simulink model "PraktikumSDR"  (R2023b)
settings: Solver=VariableStepAuto  StartTime=0.0  StopTime=19200*Ts  RelTol=1e-3
model workspace (MAT data in the model file):
  CodeRate = 0.75
  M = 16
  PunctureVector = [1; 1; 0; 1; 0; 1]
  TracebackDepth = 48
  Trelli.numInputSymbols = 2
  Trelli.numOutputSymbols = 4
  Trelli.numStates = 64
  Trelli.nextStates = [0  32; 0  32; 1  33; 1  33; 2  34; 2  34; 3  35; 3  35; 4  36; 4  36; 5  37; 5  37; 6  38; 6  38; 7  39; 7  39; 8  40; 8  40; 9  41; 9  41; 10  42; 10  42; 11  43; 11  43; 12  44; 12  44; 13  45; 13  45; 14  46; 14  46; 15  47; 15  47; 16  48; 16  48; 17  49; 17  49; 18  50; 18  50; 19  51; 19  51; 20  52; 20  52; 21  53; 21  53; 22  54; 22  54; 23  55; 23  55; 24  56; 24  56; 25  57; 25  57; 26  58; 26  58; 27  59; 27  59; 28  60; 28  60; 29  61; 29  61; 30  62; 30  62; 31  63; 31  63]
  Trelli.outputs = [0  3; 3  0; 1  2; 2  1; 0  3; 3  0; 1  2; 2  1; 3  0; 0  3; 2  1; 1  2; 3  0; 0  3; 2  1; 1  2; 3  0; 0  3; 2  1; 1  2; 3  0; 0  3; 2  1; 1  2; 0  3; 3  0; 1  2; 2  1; 0  3; 3  0; 1  2; 2  1; 2  1; 1  2; 3  0; 0  3; 2  1; 1  2; 3  0; 0  3; 1  2; 2  1; 0  3; 3  0; 1  2; 2  1; 0  3; 3  0; 1  2; 2  1; 0  3; 3  0; 1  2; 2  1; 0  3; 3  0; 2  1; 1  2; 3  0; 0  3; 2  1; 1  2; 3  0; 0  3]
  Ts = 5e-08
undefined symbols (not defined in the file or in its folder): doppler, get, gray, hot, j, magnitude
libraries: dspxfrm3 x12, dspobslib x11, dspstat3 x10, dspsigops x10, dspindex x7, commrflib2 x6, commcnvcod2 x6, commdigbbndam3 x6, simulink x6, commchan3 x4, dspquant2 x4, commsink2 x4
(part 1 of 3)
settings Model: Creator=suttarar@hu-berlin.de  LastModifiedBy=suttarar@hu-berlin.de

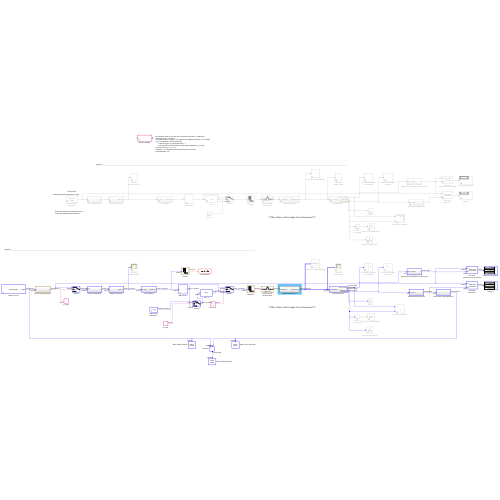
[thumbnail: Simulink's stored preview of the top-level diagram]
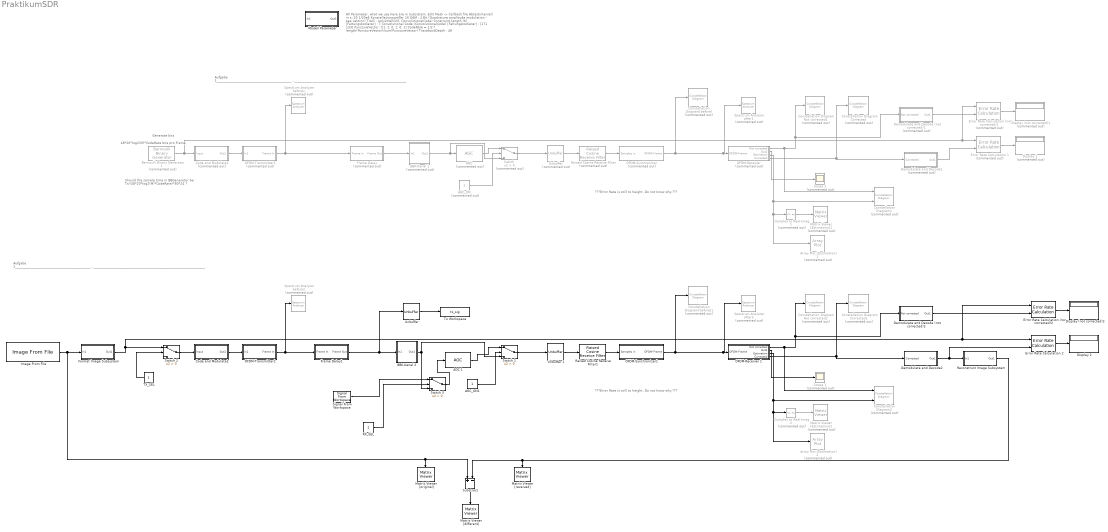
== system PraktikumSDR ==
  note: ???Error Rate is still to height. Do not know why.???
  note: Aufgabe 1______________________________________________________________________________________________________________________________________________________________________________________________________________________________________________________________________________________________________________
  note: Should the sample time in BBGenerator be:
      | Ts/(48*20*log2(M)*CodeRate)*80*24 ?
  note: All Parameter, what we use here are in Subsistem. Edit Mask -> Callback file
      | Abtastintervall in s: 20 1/20e6
      | Konstellationsgröße: 16 QAM : 4 Bit (Quadrature amplitude modulation - see Lektion)
      | Trelli : poly2trellis(K, ConvolutionalCode)
      | Constraint length (K) [Faltungskodierer] : 7
      | Convolutional Code (ConvolutionalCode) [Faltungskodierer] : [171 133]
      | PunctureVector: [[1; 1; 0; 1; 0; 1]
      | CodeRate = 1/2 * length(PunctureVector)/sum(PunctureVector)
      | TracebackDepth : 48
  note: 48*20*log2(M)*CodeRate bits pro Frame
  note: Generate bits
  note: ???Error Rate is still to height. Do not know why.???
  note: Aufgabe 2______________________________________________________________________________________________________________________________________________________________________________________________________________________________________________________________________________________________________________
  "AGC " : commrfcorlib/AGC  Commented=on  LegacyMode=off  DetectorMethod=Rectifier  LoopMethod=Linear  UpdatePeriod=100  StepSize=0.1  AdaptationStepSize=0.01  DesiredOutputPower=1  AveragingLength=16  MaximumGain=30  MaxPowerGain=10  GainOutputPort=off  InputPowerOutputPort=off  SimulateUsing=Interpreted execution
  AGC 1 : commrfcorlib/AGC  LegacyMode=off  DetectorMethod=Rectifier  LoopMethod=Linear  UpdatePeriod=100  StepSize=0.1  AdaptationStepSize=0.5  DesiredOutputPower=1  AveragingLength=16  MaximumGain=30  MaxPowerGain=10  GainOutputPort=off  InputPowerOutputPort=off  SimulateUsing=Interpreted execution
  AGC_ON : Constant  Commented=on
  AGC_ON1 : Constant
  Array Plot [Estimation]1 : ArrayPlot  Commented=on  WindowPosition=[886.000000,184.000000,800.000000,500.000000,]  ScopeFrameLocation=window  PlotAsMagnitudePhase=on  YLimits=[-0.4803 1.494]
  Array Plot [Estimation]2 : ArrayPlot  Commented=on  WindowPosition=[886.000000,184.000000,800.000000,500.000000,]  ScopeFrameLocation=window  PlotAsMagnitudePhase=on  YLimits=[-0.4803 1.494]
  BBK-Kanal 1 : Subsystem  Commented=on  mask{MaxDoppler=20, PathDelays=[0 2 5].*Ts, PathGains=[0 -16 -24], EnableMultipath=1, PathLoss=0, FrequencyOffset=50000, PhaseOffset=0, SNR=25}
      mask prompts: MaxDoppler "Dopplerverschiebung"; PathDelays "Pfadverzoergerungen"; PathGains "Pfadverstaerkungen"; EnableMultipath "SwitchBlock"; PathLoss "Pfadverlust"; FrequencyOffset "Frequenzverschiebung"; PhaseOffset "Phasenverschiebung"; SNR "AWG-Rauschen"
  BBK-Kanal 2 : Subsystem  mask{MaxDoppler=20, PathDelays=[0 2 5].*Ts, PathGains=[0 -16 -24], EnableMultipath=1, PathLoss=0, FrequencyOffset=50000, PhaseOffset=0, SNR=15}
      mask prompts: MaxDoppler "Dopplerverschiebung"; PathDelays "Pfadverzoergerungen"; PathGains "Pfadverstaerkungen"; EnableMultipath "SwitchBlock"; PathLoss "Pfadverlust"; FrequencyOffset "Frequenzverschiebung"; PhaseOffset "Phasenverschiebung"; SNR "AWG-Rauschen"
  Bernoulli Binary Generator 1 : commrandsrc3/Bernoulli Binary Generator  Commented=on  ProbabilityOfZero=0.5  SeedSource=Auto  Seed=0  SampleTime=Ts/(48*20*log2(M)*CodeRate)*80*24  SamplesPerFrame=48*20*log2(M)*CodeRate  OutputDataType=double  SimulateUsing=Interpreted execution
  Code and Modulate1 : Subsystem  Commented=on
  Code and Modulate2 : Subsystem
  Complex to Real-Imag 1 : ComplexToRealImag  Commented=on  Output=Real
  Complex to Real-Imag 2 : ComplexToRealImag  Commented=on  Output=Real
  Constellation Diagram Corrected : ConstellationDiagram  Commented=on  WindowPosition=[869.000000,188.000000,600.000000,600.000000,]  ScopeFrameLocation=window  SymbolsToDisplaySource=Property  SymbolsToDisplay=500  ReferenceConstellation="[0.70711+0.70711i        -0.70711+0.70711i        -0.70711-0.70711i         0.70711-0.70711i]"  XLimits=[-1.71,1.66]  YLimits=[-1.67,1.51]  ShowLegend=on
  Constellation Diagram Corrected1 : ConstellationDiagram  Commented=on  WindowPosition=[869.000000,188.000000,600.000000,600.000000,]  ScopeFrameLocation=window  SymbolsToDisplaySource=Property  SymbolsToDisplay=500  ReferenceConstellation="[0.70711+0.70711i        -0.70711+0.70711i        -0.70711-0.70711i         0.70711-0.70711i]"  XLimits=[-1.71,1.66]  YLimits=[-1.67,1.51]  ShowLegend=on
  Constellation Diagram Not corrected1 : ConstellationDiagram  Commented=on  WindowPosition=[922.000000,306.000000,600.000000,600.000000,]  ScopeFrameLocation=window  ReferenceConstellation="[0.70711+0.70711i        -0.70711+0.70711i        -0.70711-0.70711i         0.70711-0.70711i]"  XLimits=[-1.55,1.51]  YLimits=[-1.43,1.46]  ShowLegend=on
  Constellation Diagram Not corrected2 : ConstellationDiagram  Commented=on  WindowPosition=[922.000000,306.000000,600.000000,600.000000,]  ScopeFrameLocation=window  ReferenceConstellation="[0.70711+0.70711i        -0.70711+0.70711i        -0.70711-0.70711i         0.70711-0.70711i]"  XLimits=[-1.55,1.51]  YLimits=[-1.43,1.46]  ShowLegend=on
  Constellation Diagram1 : ConstellationDiagram  Commented=on  NumInputPorts=2  WindowPosition=[1234.000000,143.000000,600.000000,600.000000,]  ScopeFrameLocation=window  ReferenceConstellation="{[0.70711+0.70711i        -0.70711+0.70711i        -0.70711-0.70711i         0.70711-0.70711i][0.70711+0.70711i        -0.70711+0.70711i        -0.70711-0.70711i         0.70711-0.70711i]}"  XLimits=[-1.55,1.51]  YLimits=[-1.43,1.46]  ShowLegend=on
  Constellation Diagram2 : ConstellationDiagram  Commented=on  NumInputPorts=2  WindowPosition=[1234.000000,143.000000,600.000000,600.000000,]  ScopeFrameLocation=window  ReferenceConstellation="{[0.70711+0.70711i        -0.70711+0.70711i        -0.70711-0.70711i         0.70711-0.70711i][0.70711+0.70711i        -0.70711+0.70711i        -0.70711-0.70711i         0.70711-0.70711i]}"  XLimits=[-1.55,1.51]  YLimits=[-1.43,1.46]  ShowLegend=on
  Constellation Diagram[before] : ConstellationDiagram  Commented=on  WindowPosition=[219.000000,183.000000,600.000000,600.000000,]  ScopeFrameLocation=window  SymbolsToDisplaySource=Property  SymbolsToDisplay=500  ReferenceConstellation="[0.70711+0.70711i        -0.70711+0.70711i        -0.70711-0.70711i         0.70711-0.70711i]"  XLimits=[-1.71,1.66]  YLimits=[-1.67,1.51]  ShowLegend=on
  Constellation Diagram[before]1 : ConstellationDiagram  Commented=on  WindowPosition=[219.000000,183.000000,600.000000,600.000000,]  ScopeFrameLocation=window  SymbolsToDisplaySource=Property  SymbolsToDisplay=500  ReferenceConstellation="[0.70711+0.70711i        -0.70711+0.70711i        -0.70711-0.70711i         0.70711-0.70711i]"  XLimits=[-1.71,1.66]  YLimits=[-1.67,1.51]  ShowLegend=on
  Demodulate and Decode (not corrected)1 : Subsystem  Commented=on
  Demodulate and Decode (not corrected)2 : Subsystem
  Demodulate and Decode1 : Subsystem  Commented=on
  Demodulate and Decode2 : Subsystem
  Display (not corrected)1 : Display  Commented=on
  Display (not corrected)2 : Display
  Display 1 : Display  Commented=on
  Display 2 : Display
  Error Rate Calculation (not corrected)1 : commsink2/Error Rate Calculation  Commented=on  N=TracebackDepth  st_delay=48*20*log2(M)*CodeRate  cp_mode=Entire frame  subframe=[]  PMode=Port  WsName=ErrorVec  RsMode2=off  stop=off  numErr=100  maxBits=1e6
  Error Rate Calculation (not corrected)2 : commsink2/Error Rate Calculation  N=TracebackDepth  st_delay=48*20*log2(M)*CodeRate  cp_mode=Entire frame  subframe=[]  PMode=Port  WsName=ErrorVec  RsMode2=off  stop=off  numErr=100  maxBits=1e6
  Error Rate Calculation 1 : commsink2/Error Rate Calculation  Commented=on  N=TracebackDepth+2880  st_delay=0  cp_mode=Entire frame  subframe=[]  PMode=Port  WsName=ErrorVec  RsMode2=off  stop=off  numErr=100  maxBits=1e6
  Error Rate Calculation 2 : commsink2/Error Rate Calculation  N=TracebackDepth+2880  st_delay=0  cp_mode=Entire frame  subframe=[]  PMode=Port  WsName=ErrorVec  RsMode2=off  stop=off  numErr=100  maxBits=1e6
  Format Image Subsystem : Subsystem
  Frame Delay : Subsystem  Commented=on
  Frame Delay1 : Subsystem
  Image From File : visionsources/Image From File  Tag=vipblks_nd  FileName=/vol/cs-hu/suttarar/hu-home/simulink_bbk/Praktikum12/Praktikum12_Dateien (1)/grayscale.jpg  Ts=2880*10*Ts/(48*20*log2(M)*CodeRate)*80*24  imagePorts=One multidimensional signal  OutPortLabels=R|G|B  ImageDataType=Inherit from input image  sdImageDataType=uint(8)  Signed=on  WordLength=16  FractionLengthMode=User-defined  FractionLength=15
  Matrix Viewer [Estimation]1 : dspobslib/Matrix Viewer  Commented=on  ImageParams=off  CMapStr=gray(256)  AxisColorbar=on  AxisParams=off  AxisOrigin=Upper left corner  AxisTickMode=Auto  XTickRange=[0 1]  YTickRange=[0 1]  XLabel=X-axis  YLabel=Y-axis  ZLabel=Z-axis  FigPos=get(0,'defaultfigureposition')  AxisZoom=off
      settings: YMin=0.99546  YMax=1.0044
  Matrix Viewer [Estimation]2 : dspobslib/Matrix Viewer  Commented=on  ImageParams=off  CMapStr=gray(256)  AxisColorbar=on  AxisParams=off  AxisOrigin=Upper left corner  AxisTickMode=Auto  XTickRange=[0 1]  YTickRange=[0 1]  XLabel=X-axis  YLabel=Y-axis  ZLabel=Z-axis  FigPos=get(0,'defaultfigureposition')  AxisZoom=off
      settings: YMin=0.99546  YMax=1.0044
  Matrix Viewer [different] : dspobslib/Matrix Viewer  ImageParams=off  CMapStr=gray(256)  AxisColorbar=on  AxisParams=off  AxisOrigin=Upper left corner  AxisTickMode=Auto  XTickRange=[0 1]  YTickRange=[0 1]  XLabel=X-axis  YLabel=Y-axis  ZLabel=Z-axis  FigPos=get(0,'defaultfigureposition')  AxisZoom=off
      settings: YMin=0  YMax=255
  Matrix Viewer [original] : dspobslib/Matrix Viewer  ImageParams=off  CMapStr=gray(256)  AxisColorbar=on  AxisParams=off  AxisOrigin=Upper left corner  AxisTickMode=Auto  XTickRange=[0 1]  YTickRange=[0 1]  XLabel=X-axis  YLabel=Y-axis  ZLabel=Z-axis  FigPos=get(0,'defaultfigureposition')  AxisZoom=off
      settings: YMin=0  YMax=255
  Matrix Viewer [received] : dspobslib/Matrix Viewer  ImageParams=off  CMapStr=gray(256)  AxisColorbar=on  AxisParams=off  AxisOrigin=Upper left corner  AxisTickMode=Auto  XTickRange=[0 1]  YTickRange=[0 1]  XLabel=X-axis  YLabel=Y-axis  ZLabel=Z-axis  FigPos=get(0,'defaultfigureposition')  AxisZoom=off
      settings: YMin=0  YMax=255
  Modell Parameter : Subsystem  mask{Ts=1/20e6, M=16, Trelli=poly2trellis(7, [171 133]), PunctureVector=[1; 1; 0; 1; 0; 1], CodeRate=0.75, TracebackDepth=48}
      mask prompts: Ts "Abtastintervall in s"; M "Konstellationsgröße"
  "OFDM-Receiver " : Subsystem  Commented=on
  OFDM-Receiver 1 : Subsystem
  OFDM-Synchronizer : Subsystem  Commented=on
  OFDM-Synchronizer1 : Subsystem
  OFDM-Transmitter1 : Subsystem  Commented=on
  OFDM-Transmitter2 : Subsystem
  RX_SEL : Constant
  Raised Cosine Receive Filter : commfilt2/Raised Cosine Receive Filter  Commented=on  filtType=Square root  R=0.2  filtSpan=10  N=2  downFactor=2  downOffset=0  filterGain=1  RateOptions=Allow multirate processing  framing=Mute  checkCoeff=off  variableName=rcRxFilt  currentFiltSpan=10  D=5  inputOffset=0  sampMode=Mute  saveAsFlag=0  rateMode=Downsampling  checkGain=Normalized  launchFVT=on  roundingMode=Floor  overflowMode=off  coeffDataTypeStr=Inherit: Same word length as input  coeffMin=[]  coeffMax=[]  coeffLastDataTypeStr=Inherit: Same word length as input  accumDataTypeStr=Inherit: Same as product output  accumLastDataTypeStr=Inherit: Same as product output  outputDataTypeStr=Inherit: Same as accumulator  outputMin=[]  outputMax=[]  outputLastDataTypeStr=Inherit: Same as accumulator
      settings: LibrarySourceBlock=|
      | commhdlfilt/Raised Cosine
      | Receive Filter
  Raised Cosine Receive Filter1 : commfilt2/Raised Cosine Receive Filter  filtType=Square root  R=0.2  filtSpan=10  N=2  downFactor=2  downOffset=0  filterGain=1  RateOptions=Allow multirate processing  framing=Mute  checkCoeff=off  variableName=rcRxFilt1  currentFiltSpan=10  D=5  inputOffset=0  sampMode=Mute  saveAsFlag=0  rateMode=Downsampling  checkGain=Normalized  launchFVT=on  roundingMode=Floor  overflowMode=off  coeffDataTypeStr=Inherit: Same word length as input  coeffMin=[]  coeffMax=[]  coeffLastDataTypeStr=Inherit: Same word length as input  accumDataTypeStr=Inherit: Same as product output  accumLastDataTypeStr=Inherit: Same as product output  outputDataTypeStr=Inherit: Same as accumulator  outputMin=[]  outputMax=[]  outputLastDataTypeStr=Inherit: Same as accumulator
      settings: LibrarySourceBlock=|
      | commhdlfilt/Raised Cosine
      | Receive Filter
  Reconstruct Image Subsystem : Subsystem
  Scope 1 : Scope  Commented=on
  Scope 2 : Scope  Commented=on
  Signal From Workspace : dspsrcs4/Signal From Workspace  X=rx_sig  Ts=Ts/4  nsamps=7680  OutputAfterFinalValue=Setting to zero  ignoreOrWarnInputAndFrameLengths=off  OutputFrames=off
  Spectrum Analyzer after1 : SpectrumAnalyzer  Commented=on  WindowPosition=[940.000000,172.000000,800.000000,500.000000,]  ScopeFrameLocation=window  Span=20000000  StartFrequency=-10000000  StopFrequency=10000000  YLimits=[-26.81296668,18.83014348]
  Spectrum Analyzer after2 : SpectrumAnalyzer  Commented=on  WindowPosition=[940.000000,172.000000,800.000000,500.000000,]  Visible=on  ScopeFrameLocation=window  Span=20000000  StartFrequency=-10000000  StopFrequency=10000000  YLimits=[-28.40563685,17.66109951]
  Spectrum Analyzer before1 : SpectrumAnalyzer  Commented=on  WindowPosition=[6.000000,502.000000,800.000000,500.000000,]  ScopeFrameLocation=window  Span=20000000  StartFrequency=-10000000  StopFrequency=10000000  YLimits=[-24.45122434,14.99996905]
  Spectrum Analyzer before2 : SpectrumAnalyzer  Commented=on  WindowPosition=[-21.000000,360.000000,800.000000,500.000000,]  ScopeFrameLocation=window  Span=20000000  StartFrequency=-10000000  StopFrequency=10000000  YLimits=[-26.72428692,14.41237789]
  Substract : Sum  Inputs=+-
  "Switch " : Switch  Commented=on  Criteria=u2 > Threshold  SaturateOnIntegerOverflow=off  InputSameDT=off
  Switch 1 : Switch  Criteria=u2 > Threshold  SaturateOnIntegerOverflow=off  InputSameDT=off
  Switch 2 : Switch  Criteria=u2 > Threshold  SaturateOnIntegerOverflow=off  InputSameDT=off
  Switch 3 : Switch  Criteria=u2 > Threshold  SaturateOnIntegerOverflow=off  InputSameDT=off
  TX_SEL : Constant
  To Workspace : ToWorkspace  VariableName=tx_sig  SampleTime=-1
      settings: MaxDataPoints=76800  Save2DSignal=2-D array (concatenate along first dimension)
  Unbuffer : Unbuffer
  "Unbuffer " : Unbuffer  Commented=on
  Unbuffer 1 : Unbuffer
  wires:
  "OFDM-Receiver "/1(Not corrected) -> Constellation Diagram1/1, Demodulate and Decode (not corrected)1/1(Not corrected), Constellation Diagram Not corrected1/1
  Code and Modulate1/1(Out1) -> OFDM-Transmitter1/1(In1)
  Complex to Real-Imag 1/1 -> Matrix Viewer [Estimation]1/1
  "OFDM-Receiver "/2(Out2) -> Scope 2/1
  "OFDM-Receiver "/4(Corrected) -> Demodulate and Decode1/1(Corrected), Constellation Diagram Corrected/1
  Error Rate Calculation 1/1 -> Display 1/1
  Error Rate Calculation (not corrected)1/1 -> Display (not corrected)1/1
  Demodulate and Decode (not corrected)1/1(Out1) -> Error Rate Calculation (not corrected)1/2
  Demodulate and Decode1/1(Out1) -> Error Rate Calculation 1/2
  Bernoulli Binary Generator 1/1 -> Error Rate Calculation (not corrected)1/1, Error Rate Calculation 1/1, Code and Modulate1/1(Input)
  "OFDM-Receiver "/3(Estimation) -> Constellation Diagram1/2, Array Plot [Estimation]1/1, Complex to Real-Imag 1/1
  BBK-Kanal 1/1(Out1) -> "Switch "/3, "AGC "/1
  "Switch "/1 -> "Unbuffer "/1
  "AGC "/1 -> "Switch "/1
  AGC_ON/1 -> "Switch "/2
  OFDM-Synchronizer/1(OFDM-Frame) -> Spectrum Analyzer after1/1, "OFDM-Receiver "/1(OFDM-Frame), Constellation Diagram[before]/1
  "Unbuffer "/1 -> Raised Cosine Receive Filter/1
  Frame Delay/1(Frame Out) -> BBK-Kanal 1/1(In1)
  Raised Cosine Receive Filter/1 -> OFDM-Synchronizer/1(Samples in)
  OFDM-Transmitter1/1(Frame In) -> Frame Delay/1(Frame In), Spectrum Analyzer before1/1
  AGC 1/1 -> Switch 1/1
  Error Rate Calculation 2/1 -> Display 2/1
  Frame Delay1/1(Frame Out) -> Unbuffer/1, BBK-Kanal 2/1(In1)
  OFDM-Receiver 1/2(Out2) -> Scope 1/1
  Raised Cosine Receive Filter1/1 -> OFDM-Synchronizer1/1(Samples in)
  OFDM-Receiver 1/1(Not corrected) -> Constellation Diagram2/1, Demodulate and Decode (not corrected)2/1(Not corrected), Constellation Diagram Not corrected2/1
  OFDM-Receiver 1/4(Corrected) -> Demodulate and Decode2/1(Corrected), Constellation Diagram Corrected1/1
  Code and Modulate2/1(Out1) -> OFDM-Transmitter2/1(In1)
  OFDM-Receiver 1/3(Estimation) -> Constellation Diagram2/2, Array Plot [Estimation]2/1, Complex to Real-Imag 2/1
  Demodulate and Decode (not corrected)2/1(Out1) -> Error Rate Calculation (not corrected)2/2
  Error Rate Calculation (not corrected)2/1 -> Display (not corrected)2/1
  OFDM-Transmitter2/1(Frame In) -> Frame Delay1/1(Frame In), Spectrum Analyzer before2/1
  BBK-Kanal 2/1(Out1) -> Switch 3/3, Switch 1/3
  Demodulate and Decode2/1(Out1) -> Reconstruct Image Subsystem/1(In1), Error Rate Calculation 2/2
  Complex to Real-Imag 2/1 -> Matrix Viewer [Estimation]2/1
  AGC_ON1/1 -> Switch 1/2
  OFDM-Synchronizer1/1(OFDM-Frame) -> Spectrum Analyzer after2/1, OFDM-Receiver 1/1(OFDM-Frame), Constellation Diagram[before]1/1
  Switch 1/1 -> Unbuffer 1/1
  Unbuffer 1/1 -> Raised Cosine Receive Filter1/1
  Substract/1 -> Matrix Viewer [different]/1
  Format Image Subsystem/1(Out1) -> Switch 2/1, Error Rate Calculation (not corrected)2/1, Error Rate Calculation 2/1
  TX_SEL/1 -> Switch 2/2
  Switch 2/1 -> Code and Modulate2/1(Input)
  Image From File/1 -> Substract/1, Matrix Viewer [original]/1, Format Image Subsystem/1(In1)
  Reconstruct Image Subsystem/1(Out1) -> Substract/2, Matrix Viewer [received]/1
  Unbuffer/1 -> To Workspace/1
  Signal From Workspace/1 -> Switch 3/1
  RX_SEL/1 -> Switch 3/2
  Switch 3/1 -> AGC 1/1

== system PraktikumSDR/BBK-Kanal 1 ==
  In1 : Inport
  AWGN Channel : commchan3/AWGN Channel  LegacyMode=off  NoiseMethod="Signal to noise ratio  (SNR)"  noiseMode="Signal to noise ratio  (SNR)"  EbNo=10  EsNo=10  SNR=SNR  BitsPerSymbol=1  SignalPower=1  SamplesPerSymbol=1  SymbolPeriod=1  VarianceSource=Parameter  Variance=1  RandomStream=Global stream  Seed=67  SimulateUsing=Code generation
  Constant : Constant  Value=EnableMultipath
  Free Space Path Loss : commrflib2/Free Space Path Loss  mode=Decibels  dB=PathLoss  d=0.100  fc=1920
  Phase/ Frequency Offset : commrflib2/Phase// Frequency Offset  phaseOffset=PhaseOffset  freqPort=off  freqOffset=FrequencyOffset
      settings: LibrarySourceBlock=|
      | commrfcorlib/Phase//
      | Frequency
      | Offset
  SISO Fading Channel : commchan3/SISO Fading Channel  InheritSampleRate=on  SampleRate=1  PathDelays=PathDelays  AveragePathGains=PathGains  NormalizePathGains=on  FadingDistribution=Rayleigh  KFactor=3  DirectPathDopplerShift=0  DirectPathInitialPhase=0  MaximumDopplerShift=MaxDoppler  DopplerSpectrum=doppler('Jakes')  RandomStream=mt19937ar with seed  Seed=73  PathGainsOutputPort=off  ChannelFilterDelayOutputPort=off  SimulateUsing=Interpreted execution  Visualization=Off  PathsForDopplerDisplay=1  SamplesToDisplay=25%
  Switch : Switch  Criteria=u2 > Threshold  SaturateOnIntegerOverflow=off  InputSameDT=off
  Out1 : Outport
  wires:
  Phase/ Frequency Offset/1 -> AWGN Channel/1
  Free Space Path Loss/1 -> Phase/ Frequency Offset/1
  AWGN Channel/1 -> Out1/1
  Switch/1 -> Free Space Path Loss/1
  SISO Fading Channel/1 -> Switch/1
  In1/1 -> Switch/3, SISO Fading Channel/1
  Constant/1 -> Switch/2

== system PraktikumSDR/BBK-Kanal 2 ==
  In1 : Inport
  AWGN Channel : commchan3/AWGN Channel  LegacyMode=off  NoiseMethod="Signal to noise ratio  (SNR)"  noiseMode="Signal to noise ratio  (SNR)"  EbNo=10  EsNo=10  SNR=SNR  BitsPerSymbol=1  SignalPower=1  SamplesPerSymbol=1  SymbolPeriod=1  VarianceSource=Parameter  Variance=1  RandomStream=Global stream  Seed=67  SimulateUsing=Code generation
  Constant : Constant  Value=EnableMultipath
  Free Space Path Loss : commrflib2/Free Space Path Loss  mode=Decibels  dB=PathLoss  d=0.100  fc=1920
  Phase/ Frequency Offset : commrflib2/Phase// Frequency Offset  phaseOffset=PhaseOffset  freqPort=off  freqOffset=FrequencyOffset
      settings: LibrarySourceBlock=|
      | commrfcorlib/Phase//
      | Frequency
      | Offset
  SISO Fading Channel : commchan3/SISO Fading Channel  InheritSampleRate=on  SampleRate=1  PathDelays=PathDelays  AveragePathGains=PathGains  NormalizePathGains=on  FadingDistribution=Rayleigh  KFactor=3  DirectPathDopplerShift=0  DirectPathInitialPhase=0  MaximumDopplerShift=MaxDoppler  DopplerSpectrum=doppler('Jakes')  RandomStream=mt19937ar with seed  Seed=73  PathGainsOutputPort=off  ChannelFilterDelayOutputPort=off  SimulateUsing=Interpreted execution  Visualization=Off  PathsForDopplerDisplay=1  SamplesToDisplay=25%
  Switch : Switch  Criteria=u2 > Threshold  SaturateOnIntegerOverflow=off  InputSameDT=off
  Out1 : Outport
  wires:
  Phase/ Frequency Offset/1 -> AWGN Channel/1
  Free Space Path Loss/1 -> Phase/ Frequency Offset/1
  AWGN Channel/1 -> Out1/1
  Switch/1 -> Free Space Path Loss/1
  SISO Fading Channel/1 -> Switch/1
  In1/1 -> Switch/3, SISO Fading Channel/1
  Constant/1 -> Switch/2

== system PraktikumSDR/Code and Modulate1 ==
  note: Modulation
  note: Faltungscodierer
  Input : Inport
  "Convolutional Encoder " : commcnvcod2/Convolutional Encoder  trellis=Trelli  opMode=Continuous  DelayedResetAction=off  hasIniStPort=off  hasFinStPort=off  usePuncVector=on  punctureVector=PunctureVector  reset=Unused parameter value
  "Rectangular QAM Modulator Baseband " : commdigbbndam3/Rectangular QAM Modulator Baseband  M=M  InType=Bit  Enc=Gray  Mapping=[0:15]  PowType=Average Power  MinDist=2  AvgPow=1  PeakPow=1  Ph=0  outDtype=double  outWordLen=16  outUDDataType=sfix(16)  outFracLenMode=Best precision  outFracLen=15  outDataTypeStr=double  outLastDataTypeStr=double
  Out1 : Outport
  wires:
  "Convolutional Encoder "/1 -> "Rectangular QAM Modulator Baseband "/1
  "Rectangular QAM Modulator Baseband "/1 -> Out1/1
  Input/1 -> "Convolutional Encoder "/1

== system PraktikumSDR/Code and Modulate2 ==
  note: Modulation
  note: Faltungscodierer
  Input : Inport
  "Convolutional Encoder " : commcnvcod2/Convolutional Encoder  trellis=Trelli  opMode=Continuous  DelayedResetAction=off  hasIniStPort=off  hasFinStPort=off  usePuncVector=on  punctureVector=PunctureVector  reset=Unused parameter value
  "Rectangular QAM Modulator Baseband " : commdigbbndam3/Rectangular QAM Modulator Baseband  M=M  InType=Bit  Enc=Gray  Mapping=[0:15]  PowType=Average Power  MinDist=2  AvgPow=1  PeakPow=1  Ph=0  outDtype=double  outWordLen=16  outUDDataType=sfix(16)  outFracLenMode=Best precision  outFracLen=15  outDataTypeStr=double  outLastDataTypeStr=double
  Out1 : Outport
  wires:
  "Convolutional Encoder "/1 -> "Rectangular QAM Modulator Baseband "/1
  "Rectangular QAM Modulator Baseband "/1 -> Out1/1
  Input/1 -> "Convolutional Encoder "/1

== system PraktikumSDR/Demodulate and Decode (not corrected)1 ==
  Not corrected : Inport
  "Data Type Conversion " : DataTypeConversion  SaturateOnIntegerOverflow=off  RndMeth=Floor
  "Gain " : Gain  Gain=-1
  "Rectangular QAM Demodulator Baseband " : commdigbbndam3/Rectangular QAM Demodulator Baseband  M=M  OutType=Bit  DecType=Approximate log-likelihood ratio  VarSource=Dialog  Variance=1  Dec=Gray  Mapping=[0:15]  PowType=Average Power  MinDist=2  AvgPow=1  PeakPow=1  Ph=0  outDtype1=Inherit via internal rule  outDtype2=Inherit via internal rule  derotateFactorWordLen=16  derotateFactorDataTypeStr=Inherit: Same word length as input  derotateFactorLastDataTypeStr=Inherit: Same word length as input  denormFactorWordLen=16  denormFactorDataTypeStr=Inherit: Same word length as input  denormFactorLastDataTypeStr=Inherit: Same word length as input  prodOutWordLen=32  prodOutOverflowMode=Wrap  prodOutRoundingMode=Floor  prodOutOvFlMode=off  prodOutOvFlModeLastStrValue=off  sumWordLen=32
  "Uniform Encoder " : dspquant2/Uniform Encoder  peak=1  bits=4  otype=Unsigned integer
  "Viterbi Decoder " : commcnvcod2/Viterbi Decoder  trellis=Trelli  isPunctured=on  punctureVector=PunctureVector  erasures=off  dectype=Soft decision  nsdecb=4  runSigValErrCheck=off  tbdepth=TracebackDepth  opmode=Continuous  reset=off  delayedResetAction=off  smWordLength=16  outDataType=double
  Out1 : Outport
  wires:
  "Uniform Encoder "/1 -> "Data Type Conversion "/1
  "Gain "/1 -> "Uniform Encoder "/1
  "Data Type Conversion "/1 -> "Viterbi Decoder "/1
  "Rectangular QAM Demodulator Baseband "/1 -> "Gain "/1
  Not corrected/1 -> "Rectangular QAM Demodulator Baseband "/1
  "Viterbi Decoder "/1 -> Out1/1

== system PraktikumSDR/Demodulate and Decode (not corrected)2 ==
  Not corrected : Inport
  "Data Type Conversion " : DataTypeConversion  SaturateOnIntegerOverflow=off  RndMeth=Floor
  "Gain " : Gain  Gain=-1
  "Rectangular QAM Demodulator Baseband " : commdigbbndam3/Rectangular QAM Demodulator Baseband  M=M  OutType=Bit  DecType=Approximate log-likelihood ratio  VarSource=Dialog  Variance=1  Dec=Gray  Mapping=[0:15]  PowType=Average Power  MinDist=2  AvgPow=1  PeakPow=1  Ph=0  outDtype1=Inherit via internal rule  outDtype2=Inherit via internal rule  derotateFactorWordLen=16  derotateFactorDataTypeStr=Inherit: Same word length as input  derotateFactorLastDataTypeStr=Inherit: Same word length as input  denormFactorWordLen=16  denormFactorDataTypeStr=Inherit: Same word length as input  denormFactorLastDataTypeStr=Inherit: Same word length as input  prodOutWordLen=32  prodOutOverflowMode=Wrap  prodOutRoundingMode=Floor  prodOutOvFlMode=off  prodOutOvFlModeLastStrValue=off  sumWordLen=32
  "Uniform Encoder " : dspquant2/Uniform Encoder  peak=1  bits=4  otype=Unsigned integer
  "Viterbi Decoder " : commcnvcod2/Viterbi Decoder  trellis=Trelli  isPunctured=on  punctureVector=PunctureVector  erasures=off  dectype=Soft decision  nsdecb=4  runSigValErrCheck=off  tbdepth=TracebackDepth  opmode=Continuous  reset=off  delayedResetAction=off  smWordLength=16  outDataType=double
  Out1 : Outport
  wires:
  "Uniform Encoder "/1 -> "Data Type Conversion "/1
  "Gain "/1 -> "Uniform Encoder "/1
  "Data Type Conversion "/1 -> "Viterbi Decoder "/1
  "Rectangular QAM Demodulator Baseband "/1 -> "Gain "/1
  Not corrected/1 -> "Rectangular QAM Demodulator Baseband "/1
  "Viterbi Decoder "/1 -> Out1/1

== system PraktikumSDR/Demodulate and Decode1 ==
  Corrected : Inport
  "Data Type Conversion " : DataTypeConversion  SaturateOnIntegerOverflow=off  RndMeth=Floor
  "Gain " : Gain  Gain=-1
  "Rectangular QAM Demodulator Baseband " : commdigbbndam3/Rectangular QAM Demodulator Baseband  M=M  OutType=Bit  DecType=Approximate log-likelihood ratio  VarSource=Dialog  Variance=1  Dec=Gray  Mapping=[0:15]  PowType=Average Power  MinDist=2  AvgPow=1  PeakPow=1  Ph=0  outDtype1=Inherit via internal rule  outDtype2=Inherit via internal rule  derotateFactorWordLen=16  derotateFactorDataTypeStr=Inherit: Same word length as input  derotateFactorLastDataTypeStr=Inherit: Same word length as input  denormFactorWordLen=16  denormFactorDataTypeStr=Inherit: Same word length as input  denormFactorLastDataTypeStr=Inherit: Same word length as input  prodOutWordLen=32  prodOutOverflowMode=Wrap  prodOutRoundingMode=Floor  prodOutOvFlMode=off  prodOutOvFlModeLastStrValue=off  sumWordLen=32
  "Uniform Encoder " : dspquant2/Uniform Encoder  peak=1  bits=4  otype=Unsigned integer
  "Viterbi Decoder " : commcnvcod2/Viterbi Decoder  trellis=Trelli  isPunctured=on  punctureVector=PunctureVector  erasures=off  dectype=Soft decision  nsdecb=4  runSigValErrCheck=off  tbdepth=TracebackDepth  opmode=Continuous  reset=off  delayedResetAction=off  smWordLength=16  outDataType=double
  Out1 : Outport
  wires:
  "Uniform Encoder "/1 -> "Data Type Conversion "/1
  "Gain "/1 -> "Uniform Encoder "/1
  "Data Type Conversion "/1 -> "Viterbi Decoder "/1
  "Rectangular QAM Demodulator Baseband "/1 -> "Gain "/1
  Corrected/1 -> "Rectangular QAM Demodulator Baseband "/1
  "Viterbi Decoder "/1 -> Out1/1

== system PraktikumSDR/Demodulate and Decode2 ==
  Corrected : Inport
  "Data Type Conversion " : DataTypeConversion  SaturateOnIntegerOverflow=off  RndMeth=Floor
  "Gain " : Gain  Gain=-1
  "Rectangular QAM Demodulator Baseband " : commdigbbndam3/Rectangular QAM Demodulator Baseband  M=M  OutType=Bit  DecType=Approximate log-likelihood ratio  VarSource=Dialog  Variance=1  Dec=Gray  Mapping=[0:15]  PowType=Average Power  MinDist=2  AvgPow=1  PeakPow=1  Ph=0  outDtype1=Inherit via internal rule  outDtype2=Inherit via internal rule  derotateFactorWordLen=16  derotateFactorDataTypeStr=Inherit: Same word length as input  derotateFactorLastDataTypeStr=Inherit: Same word length as input  denormFactorWordLen=16  denormFactorDataTypeStr=Inherit: Same word length as input  denormFactorLastDataTypeStr=Inherit: Same word length as input  prodOutWordLen=32  prodOutOverflowMode=Wrap  prodOutRoundingMode=Floor  prodOutOvFlMode=off  prodOutOvFlModeLastStrValue=off  sumWordLen=32
  "Uniform Encoder " : dspquant2/Uniform Encoder  peak=1  bits=4  otype=Unsigned integer
  "Viterbi Decoder " : commcnvcod2/Viterbi Decoder  trellis=Trelli  isPunctured=on  punctureVector=PunctureVector  erasures=off  dectype=Soft decision  nsdecb=4  runSigValErrCheck=off  tbdepth=TracebackDepth  opmode=Continuous  reset=off  delayedResetAction=off  smWordLength=16  outDataType=double
  Out1 : Outport
  wires:
  "Uniform Encoder "/1 -> "Data Type Conversion "/1
  "Gain "/1 -> "Uniform Encoder "/1
  "Data Type Conversion "/1 -> "Viterbi Decoder "/1
  "Rectangular QAM Demodulator Baseband "/1 -> "Gain "/1
  Corrected/1 -> "Rectangular QAM Demodulator Baseband "/1
  "Viterbi Decoder "/1 -> Out1/1

== system PraktikumSDR/Format Image Subsystem ==
  In1 : Inport
  Buffer : Buffer  N=60*6  OutputFrames=off
  Data Type Conversion : DataTypeConversion  OutDataTypeStr=double  SaturateOnIntegerOverflow=off  RndMeth=Floor
  Integer to Bit Converter : simulink/Logic and Bit Operations/Integer to Bit Converter  nbits=8  signedInputValues=Unsigned  bitOrder=MSB first  outDtype=Inherit via internal rule
  Reshape : Reshape  OutputDimensionality=Column vector (2-D)
  Out1 : Outport
  wires:
  In1/1 -> Reshape/1
  Reshape/1 -> Buffer/1
  Buffer/1 -> Data Type Conversion/1
  Data Type Conversion/1 -> Integer to Bit Converter/1
  Integer to Bit Converter/1 -> Out1/1

== system PraktikumSDR/Frame Delay ==
  Frame In : Inport
  DELAY_ON : Constant
  "Matrix Concatenate " : Concatenate  Mode=Multidimensional array
  Raised Cosine Transmit Filter : commfilt2/Raised Cosine Transmit Filter  filtType=Square root  R=0.2  filtSpan=10  N=2  filterGain=1  InputProcessing=Columns as channels (frame based)  RateOptions=Enforce single-rate processing  framing=Mute  checkCoeff=off  variableName=rcTxFilt  checkGain=Normalized  sampMode=Mute  saveAsFlag=0  currentFiltSpan=10  D=5  launchFVT=on  roundingMode=Floor  overflowMode=off  coeffDataTypeStr=Inherit: Same word length as input  coeffMin=[]  coeffMax=[]  coeffLastDataTypeStr=Inherit: Same word length as input  outputDataTypeStr=Inherit: Same as accumulator  outputMin=[]  outputMax=[]  outputLastDataTypeStr=Inherit: Same as accumulator
      settings: LibrarySourceBlock=|
      | commhdlfilt/Raised Cosine
      | Transmit Filter
  "Random Integer Generator " : commrandsrc3/Random Integer Generator  SetSize=1920  SeedSource=Auto  Seed=0  SampleTime=Ts*80*24  SamplesPerFrame=1  OutputDataType=double  SimulateUsing=Interpreted execution
  Reshape 2 : Reshape  OutputDimensionality=Column vector (2-D)
  Spaltenvector [Zero] : Constant  Value=complex(zeros(1,1920))  VectorParams1D=off
  "Switch " : Switch  Criteria=u2 > Threshold  SaturateOnIntegerOverflow=off  InputSameDT=off
  "Variable Integer Delay " : Delay  DelayLengthSource=Input port  DelayLengthUpperLimit=1920*2  InputProcessing=Columns as channels (frame based)
      settings: InputPortMap=u0,p1
  Frame Out : Outport
  wires:
  Frame In/1 -> "Matrix Concatenate "/1
  Spaltenvector [Zero]/1 -> Reshape 2/1
  Reshape 2/1 -> "Matrix Concatenate "/2
  "Matrix Concatenate "/1 -> Raised Cosine Transmit Filter/1
  "Random Integer Generator "/1 -> "Variable Integer Delay "/2
  "Variable Integer Delay "/1 -> "Switch "/1
  DELAY_ON/1 -> "Switch "/2
  "Switch "/1 -> Frame Out/1
  Raised Cosine Transmit Filter/1 -> "Switch "/3, "Variable Integer Delay "/1

== system PraktikumSDR/Frame Delay1 ==
  Frame In : Inport
  DELAY_ON : Constant
  "Matrix Concatenate " : Concatenate  Mode=Multidimensional array
  Raised Cosine Transmit Filter : commfilt2/Raised Cosine Transmit Filter  filtType=Square root  R=0.2  filtSpan=10  N=2  filterGain=1  InputProcessing=Columns as channels (frame based)  RateOptions=Enforce single-rate processing  framing=Mute  checkCoeff=off  variableName=rcTxFilt  checkGain=Normalized  sampMode=Mute  saveAsFlag=0  currentFiltSpan=10  D=5  launchFVT=on  roundingMode=Floor  overflowMode=off  coeffDataTypeStr=Inherit: Same word length as input  coeffMin=[]  coeffMax=[]  coeffLastDataTypeStr=Inherit: Same word length as input  outputDataTypeStr=Inherit: Same as accumulator  outputMin=[]  outputMax=[]  outputLastDataTypeStr=Inherit: Same as accumulator
      settings: LibrarySourceBlock=|
      | commhdlfilt/Raised Cosine
      | Transmit Filter
  "Random Integer Generator " : commrandsrc3/Random Integer Generator  SetSize=1920  SeedSource=Auto  Seed=0  SampleTime=Ts*80*24  SamplesPerFrame=1  OutputDataType=double  SimulateUsing=Interpreted execution
  Reshape 2 : Reshape  OutputDimensionality=Column vector (2-D)
  Spaltenvector [Zero] : Constant  Value=complex(zeros(1,1920))  VectorParams1D=off
  "Switch " : Switch  Criteria=u2 > Threshold  SaturateOnIntegerOverflow=off  InputSameDT=off
  "Variable Integer Delay " : Delay  DelayLengthSource=Input port  DelayLengthUpperLimit=1920*2  InputProcessing=Columns as channels (frame based)
      settings: InputPortMap=u0,p1
  Frame Out : Outport
  wires:
  Frame In/1 -> "Matrix Concatenate "/1
  Spaltenvector [Zero]/1 -> Reshape 2/1
  Reshape 2/1 -> "Matrix Concatenate "/2
  "Matrix Concatenate "/1 -> Raised Cosine Transmit Filter/1
  "Random Integer Generator "/1 -> "Variable Integer Delay "/2
  "Variable Integer Delay "/1 -> "Switch "/1
  DELAY_ON/1 -> "Switch "/2
  "Switch "/1 -> Frame Out/1
  Raised Cosine Transmit Filter/1 -> "Switch "/3, "Variable Integer Delay "/1

== system PraktikumSDR/Modell Parameter ==
  In1 : Inport
  Out1 : Outport
  wires:
  In1/1 -> Out1/1

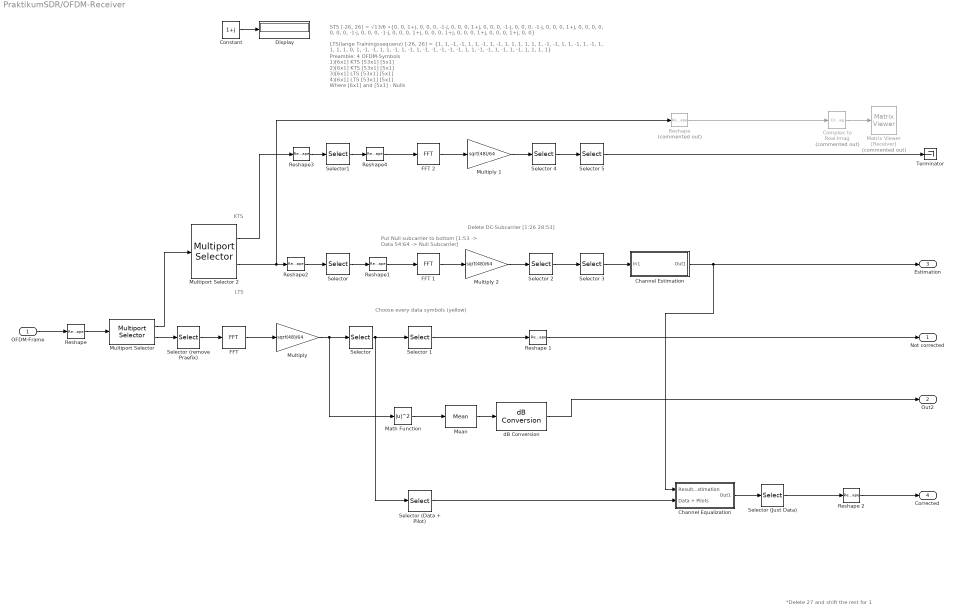
== system PraktikumSDR/OFDM-Receiver  ==
  note: *Delete 27 and shift the rest for 1
  note: Delete DC-Subcarrier [1:26 28:53]
  note: Put Null subcarrier to bottom
      | [1:53 -> Data 54:64 -> Null Subcarrier]
  note: LTS
  note: KTS
  note: Choose every data symbols (yellow)
  note: LTS(lange Trainingssequenz) [-26, 26] = {1, 1, -1, -1, 1, 1, -1, 1, -1, 1, 1, 1, 1, 1, 1, -1, -1, 1, 1, -1, 1, -1, 1, 1, 1, 1, 0, 1, -1, -1, 1, 1, -1, 1, -1, 1, -1, -1, -1, -1, -1, 1, 1, -1, -1, 1, -1, 1, -1, 1, 1, 1, 1}
  note: Preamble: 4 OFDM-Symbols
      | 1)[6x1] KTS [53x1] [5x1]
      | 2)[6x1] KTS [53x1] [5x1]
      | 3)[6x1] LTS [53x1] [5x1]
      | 4)[6x1] LTS [53x1] [5x1]
      |
      | Where [6x1] and [5x1] - Nulls
  note: STS [-26, 26] = √13/6 ∙{0, 0, 1+j, 0, 0, 0, -1-j, 0, 0, 0, 1+j, 0, 0, 0, -1-j, 0, 0, 0, -1-j, 0, 0, 0, 1+j, 0, 0, 0, 0, 0, 0, 0, -1-j, 0, 0, 0, -1-j, 0, 0, 0, 1+j, 0, 0, 0, 1+j, 0, 0, 0, 1+j, 0, 0, 0, 1+j, 0, 0}
  OFDM-Frame : Inport
  Channel Equalization : Subsystem
  Channel Estimation : Subsystem
  "Complex to Real-Imag " : ComplexToRealImag  Commented=on  Output=Real
  Constant : Constant  Value=1+j
  Display : Display
  "FFT " : dspxfrm3/FFT  FFTImplementation=Auto  CompMethod=Table lookup  TableOpt=NEW  TableOptActive=Speed  BitRevOrder=off  Normalize=off  InheritFFTLength=on  FFTLength=64  WrapInput=on  roundingMode=Floor  overflowMode=off  firstCoeffDataTypeStr=Inherit: Same word length as input  firstCoeffLastDataTypeStr=Inherit: Same word length as input  outputMin=[]  outputMax=[]
  FFT 1 : dspxfrm3/FFT  FFTImplementation=Auto  CompMethod=Table lookup  TableOpt=NEW  TableOptActive=Speed  BitRevOrder=off  Normalize=off  InheritFFTLength=on  FFTLength=64  WrapInput=on  roundingMode=Floor  overflowMode=off  firstCoeffDataTypeStr=Inherit: Same word length as input  firstCoeffLastDataTypeStr=Inherit: Same word length as input  outputMin=[]  outputMax=[]
  FFT 2 : dspxfrm3/FFT  FFTImplementation=Auto  CompMethod=Table lookup  TableOpt=NEW  TableOptActive=Speed  BitRevOrder=off  Normalize=off  InheritFFTLength=on  FFTLength=64  WrapInput=on  roundingMode=Floor  overflowMode=off  firstCoeffDataTypeStr=Inherit: Same word length as input  firstCoeffLastDataTypeStr=Inherit: Same word length as input  outputMin=[]  outputMax=[]
  "Math Function " : Math  Operator=magnitude^2
  Matrix Viewer [Receiver] : dspobslib/Matrix Viewer  Commented=on  ImageParams=off  CMapStr=gray(256)  AxisColorbar=on  AxisParams=off  AxisOrigin=Upper left corner  AxisTickMode=Auto  XTickRange=[0 1]  YTickRange=[0 1]  XLabel=X-axis  YLabel=Y-axis  ZLabel=Z-axis  FigPos=get(0,'defaultfigureposition')  AxisZoom=off
      settings: YMin=-1.4434  YMax=1.4434
  "Mean " : dspstat3/Mean  run=off  InputProcessing=Columns as channels (frame based)  reset_popup=None  directionMode=Each row  dimension=1  roiEnable=off  roiType=Rectangles  roiPortion=Entire ROI  roiOutput=Individual statistics for each ROI  roiFlag=off  roundingMode=Floor  overflowMode=off  outputDataTypeStr=Inherit: Same as accumulator  outputMin=[]  outputMax=[]  outputLastDataTypeStr=Inherit: Same as accumulator
  "Multiply " : Gain  Gain=sqrt(48)/64
  Multiply 1 : Gain  Gain=sqrt(48)/64
  Multiply 2 : Gain  Gain=sqrt(48)/64
  "Multiport Selector " : dspindex/Multiport Selector  rowsOrCols=Columns  idxCellArray={[1:4], [5:24]}  idxErrMode=Clip Index
  Multiport Selector 2 : dspindex/Multiport Selector  rowsOrCols=Columns  idxCellArray={[1:2], [3:4]}  idxErrMode=Clip Index
  Reshape : Reshape  Commented=on  OutputDimensionality=Column vector (2-D)
  "Reshape " : Reshape  OutputDimensionality=Customize  OutputDimensions=[80,24]
  Reshape 1 : Reshape  OutputDimensions=[64,24]
  Reshape 2 : Reshape  OutputDimensions=[64,24]
  Reshape1 : Reshape  OutputDimensionality=Customize  OutputDimensions=[64,2]
  Reshape2 : Reshape  OutputDimensionality=Column vector (2-D)
  Reshape3 : Reshape  OutputDimensionality=Column vector (2-D)
  Reshape4 : Reshape  OutputDimensionality=Customize  OutputDimensions=[64,2]
  Selector : Selector  NumberOfDimensions=2  InputPortWidth=3  IndexOptions=Index vector (dialog),Select all  Indices=[33:160],1  OutputSizes=1,1
  "Selector " : Selector  NumberOfDimensions=2  InputPortWidth=3  IndexOptions=Index vector (dialog),Select all  Indices=[39:64 1:38],1  OutputSizes=1,1
  Selector (remove Praefix) : Selector  NumberOfDimensions=2  InputPortWidth=3  IndexOptions=Index vector (dialog),Select all  Indices=[17:80],1  OutputSizes=1,1
  Selector (Data + Pilot) : Selector  NumberOfDimensions=2  InputPortWidth=3  IndexOptions=Index vector (dialog),Select all  Indices=[1:26 28:53],1  OutputSizes=1,1
  Selector (Just Data) : Selector  NumberOfDimensions=2  InputPortWidth=3  IndexOptions=Index vector (dialog),Select all  Indices=[1:5 7:19 21:32 34:46 48:52],1  OutputSizes=1,1
  Selector 1 : Selector  NumberOfDimensions=2  InputPortWidth=3  IndexOptions=Index vector (dialog),Select all  Indices=[1:5 7:19 21:26 28:33 35:47 49:53],1  OutputSizes=1,1
  Selector 2 : Selector  NumberOfDimensions=2  InputPortWidth=3  IndexOptions=Index vector (dialog),Select all  Indices=[39:64 1:38],1  OutputSizes=1,1
  Selector 3 : Selector  NumberOfDimensions=2  InputPortWidth=3  IndexOptions=Index vector (dialog),Select all  Indices=[1:26 28:53],1  OutputSizes=1,1
  Selector 4 : Selector  NumberOfDimensions=2  InputPortWidth=3  IndexOptions=Index vector (dialog),Select all  Indices=[39:64 1:38],1  OutputSizes=1,1
  Selector 5 : Selector  NumberOfDimensions=2  InputPortWidth=3  IndexOptions=Index vector (dialog),Select all  Indices=[1:26 28:53],1  OutputSizes=1,1
  Selector1 : Selector  NumberOfDimensions=2  InputPortWidth=3  IndexOptions=Index vector (dialog),Select all  Indices=[33:160],1  OutputSizes=1,1
  "Terminator " : Terminator
  "dB Conversion " : dspmathops/dB Conversion  dBtype=dB  intype=Power  R=1  fuzz=off
      settings: LibrarySourceBlock=commutil2/dB Conversion
  Not corrected : Outport
  Out2 : Outport  Port=2
  Estimation : Outport  Port=3
  Corrected : Outport  Port=4
  wires:
  "Mean "/1 -> "dB Conversion "/1
  "Math Function "/1 -> "Mean "/1
  "FFT "/1 -> "Multiply "/1
  OFDM-Frame/1 -> "Reshape "/1
  "Selector "/1 -> Selector (Data + Pilot)/1, Selector 1/1
  "Reshape "/1 -> "Multiport Selector "/1
  "Multiport Selector "/2 -> Selector (remove Praefix)/1
  "Multiport Selector "/1 -> Multiport Selector 2/1
  "dB Conversion "/1 -> Out2/1
  Selector 1/1 -> Reshape 1/1
  Reshape 1/1 -> Not corrected/1
  "Multiply "/1 -> "Math Function "/1, "Selector "/1
  Channel Estimation/1(Out1) -> Channel Equalization/1(Result from Channel Estimation), Estimation/1
  Selector 2/1 -> Selector 3/1
  Multiply 2/1 -> Selector 2/1
  FFT 1/1 -> Multiply 2/1
  Selector 3/1 -> Channel Estimation/1(In1)
  "Complex to Real-Imag "/1 -> Matrix Viewer [Receiver]/1
  Selector (Data + Pilot)/1 -> Channel Equalization/2(Data + Pilots)
  Channel Equalization/1(Out1) -> Selector (Just Data)/1
  Selector (Just Data)/1 -> Reshape 2/1
  Reshape 2/1 -> Corrected/1
  Selector (remove Praefix)/1 -> "FFT "/1
  Multiport Selector 2/2 -> Reshape/1, Reshape2/1
  Multiport Selector 2/1 -> Reshape3/1
  Reshape/1 -> "Complex to Real-Imag "/1
  Selector/1 -> Reshape1/1
  Reshape1/1 -> FFT 1/1
  Reshape2/1 -> Selector/1
  Constant/1 -> Display/1
  Reshape3/1 -> Selector1/1
  Selector1/1 -> Reshape4/1
  Reshape4/1 -> FFT 2/1
  FFT 2/1 -> Multiply 1/1
  Multiply 1/1 -> Selector 4/1
  Selector 4/1 -> Selector 5/1
  Selector 5/1 -> "Terminator "/1
